simulink model "system_sim"  (R2015b)
settings: Solver=ode45  StartTime=0.0  StopTime=100  RelTol=1e-3
InitFcn:
  | param
undefined symbols (not defined in the file or in its folder): ctrl, P
settings Model: Creator=beard  LastModifiedBy=magiccjae
settings DataIOCC: SaveFormat=Array  SignalLoggingSaveFormat=ModelDataLogs
settings OptimizationCC: ExpressionDepthLimit=2147483647  InitFltsAndDblsToZero=on
settings DebuggingCC: UnderspecifiedInitializationDetection=Classic  MergeDetectMultiDrivingBlocksExec=none  SolverPrmCheckMsg=warning  FcnCallInpInsideContextMsg=UseLocalSettings  StateNameClashWarn=warning
settings HardwareCC: ProdBitPerPointer=32  ProdLargestAtomicFloat=None  ProdIntDivRoundTo=Undefined  ProdEndianess=Unspecified  ProdWordSize=32  ProdHWDeviceType=32-bit Generic
settings GRTTargetCC: GeneratePreprocessorConditionals=Disable all  CombineOutputUpdateFcns=off  GRTInterface=on
settings ConfigComp: CovModelRefEnable=Off

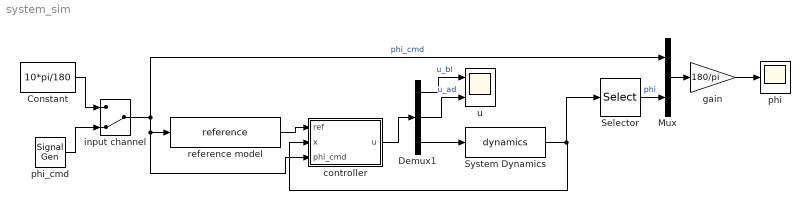
== system system_sim ==
  Constant : Constant  Value=10*pi/180
  Demux1 : Demux  Outputs=[1; 1; 1]
  Mux : Mux  Inputs=2
  Selector : Selector  InputPortWidth=2  IndexOptions=Index vector (dialog)  Indices=[1]  OutputSizes=1
  System Dynamics : S-Function  FunctionName=dynamics  Parameters=P  SFunctionDeploymentMode=off  EnableBusSupport=off
  controller : Subsystem
  gain : Gain  Gain=180/pi
  input channel : ManualSwitch  CurrentSetting=0
  phi : Scope
  phi_cmd : SignalGenerator  WaveForm=square  Amplitude=20*pi/180  Frequency=.05
  reference model : S-Function  FunctionName=reference  Parameters=P  SFunctionDeploymentMode=off  EnableBusSupport=off
  u : Scope  NumInputPorts=2
  wires:
  System Dynamics/1 -> Selector/1, controller/2(x)
  Selector/1 -> Mux/2  "phi"
  reference model/1 -> controller/1(ref)
  input channel/1 -> Mux/1, controller/3(phi_cmd), reference model/1  "phi_cmd"
  Constant/1 -> input channel/1
  phi_cmd/1 -> input channel/2
  Mux/1 -> gain/1
  gain/1 -> phi/1
  controller/1(u) -> Demux1/1
  Demux1/1 -> u/1  "u_bl"
  Demux1/2 -> u/2  "u_ad"
  Demux1/3 -> System Dynamics/1

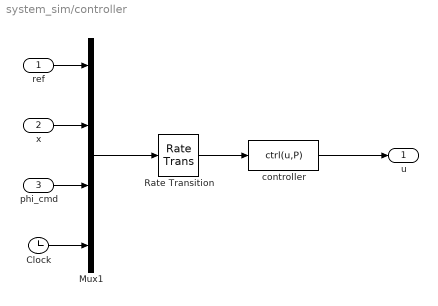
== system system_sim/controller ==
  ref : Inport
  x : Inport  Port=2
  phi_cmd : Inport  Port=3
  Clock : Clock
  Mux1 : Mux
  Rate Transition : RateTransition  OutPortSampleTime=P.Ts
  controller : MATLABFcn  MATLABFcn=ctrl(u,P)  OutputDimensions=3
  u : Outport
  wires:
  Mux1/1 -> Rate Transition/1
  ref/1 -> Mux1/1
  controller/1 -> u/1
  Rate Transition/1 -> controller/1
  x/1 -> Mux1/2
  Clock/1 -> Mux1/4
  phi_cmd/1 -> Mux1/3
